simulink library "vmc"  (R2021b)
settings: Solver=VariableStepAuto  StartTime=0.0  StopTime=10.0  RelTol=1e-3
undefined symbols (not defined in the file or in its folder): AVMC_ACCDeltaTqIGain4OVRD_X_kph, AVMC_ACCDeltaTqIGain4OVRD_Y_mps2, AVMC_ACCDeltaTqIGain_X_kph, AVMC_ACCDeltaTqIGain_Y_mps2, AVMC_ACCDeltaTqPGain_X_kph, AVMC_ACCDeltaTqPGain_Y_kph, AVMC_ACCLongSteadyCtrl_X_kph, AVMC_ADSPosGFBDeltaTq_X_kph, AVMC_ADSPosGFBDeltaTq_Y_mps2, AVMC_AggressJerkPCT4AT_X_kph, AVMC_AggressJerkPCT_X_kph, AVMC_AggressLimitPCT4AT_X_kph, AVMC_AggressLimitPCT_X_kph, AVMC_CCLongSteadyCtrl_X_kph, AVMC_DISCDeltaTqIGain_X_kph, AVMC_DISCDeltaTqIGain_Y_mps2, AVMC_DISCDeltaTqPGain_X_kph, AVMC_DISCDeltaTqPGain_Y_kph, AVMC_ESCRegenOut_X_kph, AVMC_ESCRegenOut_Y_Deg, AVMC_ESCRegenOutEnSpd_X_Deg, AVMC_ISOAccLimit_X_mps, AVMC_ISODecLimit_X_mps, AVMC_ISOJerk_X_mps, AVMC_LatESCRegenOut_X_kph, AVMC_LatESCRegenOut_Y_Deg, AVMC_LongAccDeadZone_X_kph, AVMC_LongAccFiltTsforP2_X_Gps, AVMC_MCPresBaseTq_X_bar, AVMC_MSALongSteadyCtrl_X_kph, AVMC_MSAPedalOvrd_X_kph, AVMC_MSASpdBand_X_kph, AVMC_MSATqDownEndTq_X_kph, AVMC_MSATqDownTime_X_kph, AVMC_OPDDisSlideRate_X_Deg, AVMC_OVRD2ActSR2FCMCMD_X_mps2, AVMC_PedalTqRWhlRatio_X_Nm, AVMC_PedalTqRWhlRatio_Y_gps, AVMC_PedalTqRWhlSlipGain_X_rat, AVMC_PedalTqRWhlSlipGain_Y_kph, AVMC_PedalTqRWhSTRGGain_X_deg, AVMC_PedalTqRWhSTRGGain_Y_kph, AVMC_RDCDetectTime_X_kph, AVMC_RDCDetectTime_Y_pct, AVMC_RDCEnSlideRate_X_Deg, AVMC_RearWhlTqRatio_X_Nm, AVMC_RearWhlTqRatio_Y_gps, AVMC_RearWhlTqSlipGain_X_rat, AVMC_RearWhlTqSlipGain_Y_kph, AVMC_RearWhlTqSTRGGain_X_deg, AVMC_RearWhlTqSTRGGain_Y_kph, AVMC_ReqBrkJoinDecSR_X_mps2, AVMC_SoftJerkPCT_X_kph, AVMC_SoftLimitPCT_X_kph, AVMC_StESCYaw_X_kph, AVMC_StESCYaw_Y_Deg, AVMC_StESCYawCom_X_kph, AVMC_StESCYawCom_Y_Gps, AVMC_TMSpdBaseTq_X_rpm, AVMC_VehHoldDecCtrlTime2_X_kph ... (+411)
libraries: hcu_lib x108, simulink x82, tqr x1, simulink_extras x1
(part 14 of 14)

== stateflow chart vmc/VMC/VMC/SpeedCalculation/RollingAverage ==
  state LatAccelRollingAverage
    (default) -> (junction 2) : {VVMC_RollAveCount_enum = ONE_INT}
    LatAccelRollingAverage -> (junction 2)
    (junction 2) -> (junction 3) : {VVMC_RollAve_kph = ZERO_FLOAT}
    (junction 3) -> (junction 100) [order 1] : [VVMC_RollAveCount_enum < KVMC_RollAveLevel_enum]
    (junction 3) -> (junction 37) [order 2]
    (junction 100) -> (junction 5) : {% Memory
        |  VVMC_Memory_raw32[VVMC_RollAveCount_enum] = VINP_RawData_kph;
        |
        |  % Memory Shift Counter
        |  VVMC_ShiftCount_enum = ONE_INT}
    (junction 5) -> (junction 7) [order 2]
    (junction 5) -> (junction 6) [order 1] : [VVMC_ShiftCount_enum <= VVMC_RollAveCount_enum]
    (junction 7) -> (junction 8) : {% Rolling Average
        |  VVMC_RollAve_kph = VVMC_RollAve_kph / VVMC_RollAveCount_enum;
        |
        |  % Rolling Average Counter
        |  VVMC_RollAveCount_enum++}
    (junction 35) -> (junction 5) : {VVMC_ShiftCount_enum++}
    (junction 6) -> (junction 36) : {% Rolling Average Sum
        |  VVMC_RollAve_kph = VVMC_RollAve_kph + VVMC_Memory_raw32[VVMC_ShiftCount_enum];
        |  }
    (junction 36) -> (junction 35)
    (junction 37) -> (junction 76) [order 1] : [VVMC_RollAveCount_enum == KVMC_RollAveLevel_enum]
    (junction 76) -> (junction 47)
    (junction 37) -> (junction 60) [order 2]
    (junction 78) -> (junction 76)
    (junction 47) -> (junction 30) : {% Memory
        |  VVMC_Memory_raw32[VVMC_RollAveCount_enum] = VINP_RawData_kph;
        |
        |  % Memory Shift Counter
        |  VVMC_ShiftCount_enum = ONE_INT;
        | }
    (junction 60) -> (junction 62) [order 1] : [VVMC_RollAveCount_enum > KVMC_RollAveLevel_enum]
    (junction 60) -> (junction 39) [order 2]
    (junction 62) -> (junction 66) : {VVMC_MemoryShiftCount_enum = ONE_INT}
    (junction 30) -> (junction 48) [order 2]
    (junction 30) -> (junction 22) [order 1] : [VVMC_ShiftCount_enum <= VVMC_RollAveCount_enum]
    (junction 48) -> (junction 45) : {% Rolling Average
        |  VVMC_RollAve_kph = VVMC_RollAve_kph / VVMC_RollAveCount_enum;
        |
        |  % Memory Shift Counter
        |  VVMC_ShiftCount_enum = ONE_INT}
    (junction 14) -> (junction 30) : {VVMC_ShiftCount_enum++}
    (junction 22) -> (junction 25) : {% Rolling Average Sum
        |  VVMC_RollAve_kph = VVMC_RollAve_kph + VVMC_Memory_raw32[VVMC_ShiftCount_enum]}
    (junction 66) -> (junction 82) [order 2]
    (junction 66) -> (junction 69) [order 1] : [VVMC_MemoryShiftCount_enum < VVMC_RollAveCount_enum]
    (junction 82) -> (junction 80) : {VVMC_RollAveCount_enum = KVMC_RollAveLevel_enum}
    (junction 73) -> (junction 66) : {VVMC_MemoryShiftCount_enum++}
    (junction 69) -> (junction 71) : {VVMC_Memory_raw32[VVMC_MemoryShiftCount_enum] =...
        |  VVMC_Memory_raw32[VVMC_RollAveCount_enum - KVMC_RollAveLevel_enum + VVMC_MemoryShiftCount_enum]}
    (junction 25) -> (junction 14)
    (junction 71) -> (junction 73)
    (junction 80) -> (junction 78)
    (junction 45) -> (junction 39) [order 2]
    (junction 45) -> (junction 15) [order 1] : [VVMC_ShiftCount_enum < VVMC_RollAveCount_enum]
    (junction 41) -> (junction 45) : { VVMC_ShiftCount_enum++}
    (junction 15) -> (junction 38) : {% Gy Memory Shift
        |  VVMC_Memory_raw32[VVMC_ShiftCount_enum] = VVMC_Memory_raw32[VVMC_ShiftCount_enum + ONE_INT]}
    (junction 38) -> (junction 41)
  data: KVMC_RollAveLevel_enum input uint8; VVMC_ShiftCount_enum local uint8; VVMC_RollAveCount_enum local uint8; VVMC_Memory_raw32 local single size=256; ZERO_FLOAT input single; ONE_INT input uint8; VVMC_RollAve_kph output single; VINP_RawData_kph input single; VVMC_MemoryShiftCount_enum local uint8

== stateflow chart vmc/VMC/VMC/SafetyControl/WheelSpeedRollingAverage/RollingAverage ==
  state LatAccelRollingAverage
    (default) -> (junction 2) : {VVMC_RollAveCount_enum = ONE_INT}
    LatAccelRollingAverage -> (junction 2)
    (junction 2) -> (junction 3) : {VVMC_LFWhlSpeedRollAveRaw_kph = ZERO_FLOAT}
    (junction 3) -> (junction 100) [order 1] : [VVMC_RollAveCount_enum < KVMC_WhlSpdRollAveLevel_enum]
    (junction 3) -> (junction 37) [order 2]
    (junction 100) -> (junction 5) : {% Memory
        |  VVMC_Memory_raw32[VVMC_RollAveCount_enum] = VINP_LFRawWhlSpeed_kph;
        |
        |  % Memory Shift Counter
        |  VVMC_ShiftCount_enum = ONE_INT}
    (junction 5) -> (junction 7) [order 2]
    (junction 5) -> (junction 6) [order 1] : [VVMC_ShiftCount_enum <= VVMC_RollAveCount_enum]
    (junction 7) -> (junction 8) : {% Rolling Average
        |  VVMC_LFWhlSpeedRollAveRaw_kph = VVMC_LFWhlSpeedRollAveRaw_kph / VVMC_RollAveCount_enum;
        |
        |  % Rolling Average Counter
        |  VVMC_RollAveCount_enum++}
    (junction 35) -> (junction 5) : {VVMC_ShiftCount_enum++}
    (junction 6) -> (junction 36) : {% Rolling Average Sum
        |  VVMC_LFWhlSpeedRollAveRaw_kph = VVMC_LFWhlSpeedRollAveRaw_kph + VVMC_Memory_raw32[VVMC_ShiftCount_enum];
        |  }
    (junction 36) -> (junction 35)
    (junction 37) -> (junction 76) [order 1] : [VVMC_RollAveCount_enum == KVMC_WhlSpdRollAveLevel_enum]
    (junction 76) -> (junction 47)
    (junction 37) -> (junction 60) [order 2]
    (junction 78) -> (junction 76)
    (junction 47) -> (junction 30) : {% Memory
        |  VVMC_Memory_raw32[VVMC_RollAveCount_enum] = VINP_LFRawWhlSpeed_kph;
        |
        |  % Memory Shift Counter
        |  VVMC_ShiftCount_enum = ONE_INT;
        | }
    (junction 60) -> (junction 62) [order 1] : [VVMC_RollAveCount_enum > KVMC_WhlSpdRollAveLevel_enum]
    (junction 60) -> (junction 39) [order 2]
    (junction 62) -> (junction 66) : {VVMC_MemoryShiftCount_enum = ONE_INT}
    (junction 30) -> (junction 48) [order 2]
    (junction 30) -> (junction 22) [order 1] : [VVMC_ShiftCount_enum <= VVMC_RollAveCount_enum]
    (junction 48) -> (junction 45) : {% Rolling Average
        |  VVMC_LFWhlSpeedRollAveRaw_kph = VVMC_LFWhlSpeedRollAveRaw_kph / VVMC_RollAveCount_enum;
        |
        |  % Memory Shift Counter
        |  VVMC_ShiftCount_enum = ONE_INT}
    (junction 14) -> (junction 30) : {VVMC_ShiftCount_enum++}
    (junction 22) -> (junction 25) : {% Rolling Average Sum
        |  VVMC_LFWhlSpeedRollAveRaw_kph = VVMC_LFWhlSpeedRollAveRaw_kph + VVMC_Memory_raw32[VVMC_ShiftCount_enum]}
    (junction 66) -> (junction 82) [order 2]
    (junction 66) -> (junction 69) [order 1] : [VVMC_MemoryShiftCount_enum < VVMC_RollAveCount_enum]
    (junction 82) -> (junction 80) : {VVMC_RollAveCount_enum = KVMC_WhlSpdRollAveLevel_enum}
    (junction 73) -> (junction 66) : {VVMC_MemoryShiftCount_enum++}
    (junction 69) -> (junction 71) : {VVMC_Memory_raw32[VVMC_MemoryShiftCount_enum] =...
        |  VVMC_Memory_raw32[VVMC_RollAveCount_enum - KVMC_WhlSpdRollAveLevel_enum + VVMC_MemoryShiftCount_enum]}
    (junction 25) -> (junction 14)
    (junction 71) -> (junction 73)
    (junction 80) -> (junction 78)
    (junction 45) -> (junction 39) [order 2]
    (junction 45) -> (junction 15) [order 1] : [VVMC_ShiftCount_enum < VVMC_RollAveCount_enum]
    (junction 41) -> (junction 45) : { VVMC_ShiftCount_enum++}
    (junction 15) -> (junction 38) : {% Gy Memory Shift
        |  VVMC_Memory_raw32[VVMC_ShiftCount_enum] = VVMC_Memory_raw32[VVMC_ShiftCount_enum + ONE_INT]}
    (junction 38) -> (junction 41)
  data: KVMC_WhlSpdRollAveLevel_enum input uint8; VVMC_ShiftCount_enum local uint8; VVMC_RollAveCount_enum local uint8; VVMC_Memory_raw32 local single size=256; ZERO_FLOAT input single; ONE_INT input uint8; VINP_LFRawWhlSpeed_kph input single; VVMC_MemoryShiftCount_enum local uint8; VVMC_LFWhlSpeedRollAveRaw_kph output single

== stateflow chart vmc/VMC/VMC/SafetyControl/WheelSpeedRollingAverage/RollingAverage1 ==
  state LatAccelRollingAverage
    (default) -> (junction 2) : {VVMC_RollAveCount_enum = ONE_INT}
    LatAccelRollingAverage -> (junction 2)
    (junction 2) -> (junction 3) : {VVMC_RFWhlSpeedRollAveRaw_kph = ZERO_FLOAT}
    (junction 3) -> (junction 100) [order 1] : [VVMC_RollAveCount_enum < KVMC_WhlSpdRollAveLevel_enum]
    (junction 3) -> (junction 37) [order 2]
    (junction 100) -> (junction 5) : {% Memory
        |  VVMC_Memory_raw32[VVMC_RollAveCount_enum] = VINP_RFRawWhlSpeed_kph;
        |
        |  % Memory Shift Counter
        |  VVMC_ShiftCount_enum = ONE_INT}
    (junction 5) -> (junction 7) [order 2]
    (junction 5) -> (junction 6) [order 1] : [VVMC_ShiftCount_enum <= VVMC_RollAveCount_enum]
    (junction 7) -> (junction 8) : {% Rolling Average
        |  VVMC_RFWhlSpeedRollAveRaw_kph = VVMC_RFWhlSpeedRollAveRaw_kph / VVMC_RollAveCount_enum;
        |
        |  % Rolling Average Counter
        |  VVMC_RollAveCount_enum++}
    (junction 35) -> (junction 5) : {VVMC_ShiftCount_enum++}
    (junction 6) -> (junction 36) : {% Rolling Average Sum
        |  VVMC_RFWhlSpeedRollAveRaw_kph = VVMC_RFWhlSpeedRollAveRaw_kph + VVMC_Memory_raw32[VVMC_ShiftCount_enum];
        |  }
    (junction 36) -> (junction 35)
    (junction 37) -> (junction 76) [order 1] : [VVMC_RollAveCount_enum == KVMC_WhlSpdRollAveLevel_enum]
    (junction 76) -> (junction 47)
    (junction 37) -> (junction 60) [order 2]
    (junction 78) -> (junction 76)
    (junction 47) -> (junction 30) : {% Memory
        |  VVMC_Memory_raw32[VVMC_RollAveCount_enum] = VINP_RFRawWhlSpeed_kph;
        |
        |  % Memory Shift Counter
        |  VVMC_ShiftCount_enum = ONE_INT;
        | }
    (junction 60) -> (junction 62) [order 1] : [VVMC_RollAveCount_enum > KVMC_WhlSpdRollAveLevel_enum]
    (junction 60) -> (junction 39) [order 2]
    (junction 62) -> (junction 66) : {VVMC_MemoryShiftCount_enum = ONE_INT}
    (junction 30) -> (junction 48) [order 2]
    (junction 30) -> (junction 22) [order 1] : [VVMC_ShiftCount_enum <= VVMC_RollAveCount_enum]
    (junction 48) -> (junction 45) : {% Rolling Average
        |  VVMC_RFWhlSpeedRollAveRaw_kph = VVMC_RFWhlSpeedRollAveRaw_kph / VVMC_RollAveCount_enum;
        |
        |  % Memory Shift Counter
        |  VVMC_ShiftCount_enum = ONE_INT}
    (junction 14) -> (junction 30) : {VVMC_ShiftCount_enum++}
    (junction 22) -> (junction 25) : {% Rolling Average Sum
        |  VVMC_RFWhlSpeedRollAveRaw_kph = VVMC_RFWhlSpeedRollAveRaw_kph + VVMC_Memory_raw32[VVMC_ShiftCount_enum]}
    (junction 66) -> (junction 82) [order 2]
    (junction 66) -> (junction 69) [order 1] : [VVMC_MemoryShiftCount_enum < VVMC_RollAveCount_enum]
    (junction 82) -> (junction 80) : {VVMC_RollAveCount_enum = KVMC_WhlSpdRollAveLevel_enum}
    (junction 73) -> (junction 66) : {VVMC_MemoryShiftCount_enum++}
    (junction 69) -> (junction 71) : {VVMC_Memory_raw32[VVMC_MemoryShiftCount_enum] =...
        |  VVMC_Memory_raw32[VVMC_RollAveCount_enum - KVMC_WhlSpdRollAveLevel_enum + VVMC_MemoryShiftCount_enum]}
    (junction 25) -> (junction 14)
    (junction 71) -> (junction 73)
    (junction 80) -> (junction 78)
    (junction 45) -> (junction 39) [order 2]
    (junction 45) -> (junction 15) [order 1] : [VVMC_ShiftCount_enum < VVMC_RollAveCount_enum]
    (junction 41) -> (junction 45) : { VVMC_ShiftCount_enum++}
    (junction 15) -> (junction 38) : {% Gy Memory Shift
        |  VVMC_Memory_raw32[VVMC_ShiftCount_enum] = VVMC_Memory_raw32[VVMC_ShiftCount_enum + ONE_INT]}
    (junction 38) -> (junction 41)
  data: KVMC_WhlSpdRollAveLevel_enum input uint8; VVMC_ShiftCount_enum local uint8; VVMC_RollAveCount_enum local uint8; VVMC_Memory_raw32 local single size=256; ZERO_FLOAT input single; ONE_INT input uint8; VINP_RFRawWhlSpeed_kph input single; VVMC_MemoryShiftCount_enum local uint8; VVMC_RFWhlSpeedRollAveRaw_kph output single

== stateflow chart vmc/VMC/VMC/SafetyControl/WheelSpeedRollingAverage/RollingAverage2 ==
  state LatAccelRollingAverage
    (default) -> (junction 2) : {VVMC_RollAveCount_enum = ONE_INT}
    LatAccelRollingAverage -> (junction 2)
    (junction 2) -> (junction 3) : {VVMC_LRWhlSpeedRollAveRaw_kph = ZERO_FLOAT}
    (junction 3) -> (junction 100) [order 1] : [VVMC_RollAveCount_enum < KVMC_WhlSpdRollAveLevel_enum]
    (junction 3) -> (junction 37) [order 2]
    (junction 100) -> (junction 5) : {% Memory
        |  VVMC_Memory_raw32[VVMC_RollAveCount_enum] = VINP_LRRawWhlSpeed_kph;
        |
        |  % Memory Shift Counter
        |  VVMC_ShiftCount_enum = ONE_INT}
    (junction 5) -> (junction 7) [order 2]
    (junction 5) -> (junction 6) [order 1] : [VVMC_ShiftCount_enum <= VVMC_RollAveCount_enum]
    (junction 7) -> (junction 8) : {% Rolling Average
        |  VVMC_LRWhlSpeedRollAveRaw_kph = VVMC_LRWhlSpeedRollAveRaw_kph / VVMC_RollAveCount_enum;
        |
        |  % Rolling Average Counter
        |  VVMC_RollAveCount_enum++}
    (junction 35) -> (junction 5) : {VVMC_ShiftCount_enum++}
    (junction 6) -> (junction 36) : {% Rolling Average Sum
        |  VVMC_LRWhlSpeedRollAveRaw_kph = VVMC_LRWhlSpeedRollAveRaw_kph + VVMC_Memory_raw32[VVMC_ShiftCount_enum];
        |  }
    (junction 36) -> (junction 35)
    (junction 37) -> (junction 76) [order 1] : [VVMC_RollAveCount_enum == KVMC_WhlSpdRollAveLevel_enum]
    (junction 76) -> (junction 47)
    (junction 37) -> (junction 60) [order 2]
    (junction 78) -> (junction 76)
    (junction 47) -> (junction 30) : {% Memory
        |  VVMC_Memory_raw32[VVMC_RollAveCount_enum] = VINP_LRRawWhlSpeed_kph;
        |
        |  % Memory Shift Counter
        |  VVMC_ShiftCount_enum = ONE_INT;
        | }
    (junction 60) -> (junction 62) [order 1] : [VVMC_RollAveCount_enum > KVMC_WhlSpdRollAveLevel_enum]
    (junction 60) -> (junction 39) [order 2]
    (junction 62) -> (junction 66) : {VVMC_MemoryShiftCount_enum = ONE_INT}
    (junction 30) -> (junction 48) [order 2]
    (junction 30) -> (junction 22) [order 1] : [VVMC_ShiftCount_enum <= VVMC_RollAveCount_enum]
    (junction 48) -> (junction 45) : {% Rolling Average
        |  VVMC_LRWhlSpeedRollAveRaw_kph = VVMC_LRWhlSpeedRollAveRaw_kph / VVMC_RollAveCount_enum;
        |
        |  % Memory Shift Counter
        |  VVMC_ShiftCount_enum = ONE_INT}
    (junction 14) -> (junction 30) : {VVMC_ShiftCount_enum++}
    (junction 22) -> (junction 25) : {% Rolling Average Sum
        |  VVMC_LRWhlSpeedRollAveRaw_kph = VVMC_LRWhlSpeedRollAveRaw_kph + VVMC_Memory_raw32[VVMC_ShiftCount_enum]}
    (junction 66) -> (junction 82) [order 2]
    (junction 66) -> (junction 69) [order 1] : [VVMC_MemoryShiftCount_enum < VVMC_RollAveCount_enum]
    (junction 82) -> (junction 80) : {VVMC_RollAveCount_enum = KVMC_WhlSpdRollAveLevel_enum}
    (junction 73) -> (junction 66) : {VVMC_MemoryShiftCount_enum++}
    (junction 69) -> (junction 71) : {VVMC_Memory_raw32[VVMC_MemoryShiftCount_enum] =...
        |  VVMC_Memory_raw32[VVMC_RollAveCount_enum - KVMC_WhlSpdRollAveLevel_enum + VVMC_MemoryShiftCount_enum]}
    (junction 25) -> (junction 14)
    (junction 71) -> (junction 73)
    (junction 80) -> (junction 78)
    (junction 45) -> (junction 39) [order 2]
    (junction 45) -> (junction 15) [order 1] : [VVMC_ShiftCount_enum < VVMC_RollAveCount_enum]
    (junction 41) -> (junction 45) : { VVMC_ShiftCount_enum++}
    (junction 15) -> (junction 38) : {% Gy Memory Shift
        |  VVMC_Memory_raw32[VVMC_ShiftCount_enum] = VVMC_Memory_raw32[VVMC_ShiftCount_enum + ONE_INT]}
    (junction 38) -> (junction 41)
  data: KVMC_WhlSpdRollAveLevel_enum input uint8; VVMC_ShiftCount_enum local uint8; VVMC_RollAveCount_enum local uint8; VVMC_Memory_raw32 local single size=256; ZERO_FLOAT input single; ONE_INT input uint8; VINP_LRRawWhlSpeed_kph input single; VVMC_MemoryShiftCount_enum local uint8; VVMC_LRWhlSpeedRollAveRaw_kph output single

== stateflow chart vmc/VMC/VMC/SafetyControl/WheelSpeedRollingAverage/RollingAverage3 ==
  state LatAccelRollingAverage
    (default) -> (junction 2) : {VVMC_RollAveCount_enum = ONE_INT}
    LatAccelRollingAverage -> (junction 2)
    (junction 2) -> (junction 3) : {VVMC_RRWhlSpeedRollAveRaw_kph = ZERO_FLOAT}
    (junction 3) -> (junction 100) [order 1] : [VVMC_RollAveCount_enum < KVMC_WhlSpdRollAveLevel_enum]
    (junction 3) -> (junction 37) [order 2]
    (junction 100) -> (junction 5) : {% Memory
        |  VVMC_Memory_raw32[VVMC_RollAveCount_enum] = VINP_RRRawWhlSpeed_kph;
        |
        |  % Memory Shift Counter
        |  VVMC_ShiftCount_enum = ONE_INT}
    (junction 5) -> (junction 7) [order 2]
    (junction 5) -> (junction 6) [order 1] : [VVMC_ShiftCount_enum <= VVMC_RollAveCount_enum]
    (junction 7) -> (junction 8) : {% Rolling Average
        |  VVMC_RRWhlSpeedRollAveRaw_kph = VVMC_RRWhlSpeedRollAveRaw_kph / VVMC_RollAveCount_enum;
        |
        |  % Rolling Average Counter
        |  VVMC_RollAveCount_enum++}
    (junction 35) -> (junction 5) : {VVMC_ShiftCount_enum++}
    (junction 6) -> (junction 36) : {% Rolling Average Sum
        |  VVMC_RRWhlSpeedRollAveRaw_kph = VVMC_RRWhlSpeedRollAveRaw_kph + VVMC_Memory_raw32[VVMC_ShiftCount_enum];
        |  }
    (junction 36) -> (junction 35)
    (junction 37) -> (junction 76) [order 1] : [VVMC_RollAveCount_enum == KVMC_WhlSpdRollAveLevel_enum]
    (junction 76) -> (junction 47)
    (junction 37) -> (junction 60) [order 2]
    (junction 78) -> (junction 76)
    (junction 47) -> (junction 30) : {% Memory
        |  VVMC_Memory_raw32[VVMC_RollAveCount_enum] = VINP_RRRawWhlSpeed_kph;
        |
        |  % Memory Shift Counter
        |  VVMC_ShiftCount_enum = ONE_INT;
        | }
    (junction 60) -> (junction 62) [order 1] : [VVMC_RollAveCount_enum > KVMC_WhlSpdRollAveLevel_enum]
    (junction 60) -> (junction 39) [order 2]
    (junction 62) -> (junction 66) : {VVMC_MemoryShiftCount_enum = ONE_INT}
    (junction 30) -> (junction 48) [order 2]
    (junction 30) -> (junction 22) [order 1] : [VVMC_ShiftCount_enum <= VVMC_RollAveCount_enum]
    (junction 48) -> (junction 45) : {% Rolling Average
        |  VVMC_RRWhlSpeedRollAveRaw_kph = VVMC_RRWhlSpeedRollAveRaw_kph / VVMC_RollAveCount_enum;
        |
        |  % Memory Shift Counter
        |  VVMC_ShiftCount_enum = ONE_INT}
    (junction 14) -> (junction 30) : {VVMC_ShiftCount_enum++}
    (junction 22) -> (junction 25) : {% Rolling Average Sum
        |  VVMC_RRWhlSpeedRollAveRaw_kph = VVMC_RRWhlSpeedRollAveRaw_kph + VVMC_Memory_raw32[VVMC_ShiftCount_enum]}
    (junction 66) -> (junction 82) [order 2]
    (junction 66) -> (junction 69) [order 1] : [VVMC_MemoryShiftCount_enum < VVMC_RollAveCount_enum]
    (junction 82) -> (junction 80) : {VVMC_RollAveCount_enum = KVMC_WhlSpdRollAveLevel_enum}
    (junction 73) -> (junction 66) : {VVMC_MemoryShiftCount_enum++}
    (junction 69) -> (junction 71) : {VVMC_Memory_raw32[VVMC_MemoryShiftCount_enum] =...
        |  VVMC_Memory_raw32[VVMC_RollAveCount_enum - KVMC_WhlSpdRollAveLevel_enum + VVMC_MemoryShiftCount_enum]}
    (junction 25) -> (junction 14)
    (junction 71) -> (junction 73)
    (junction 80) -> (junction 78)
    (junction 45) -> (junction 39) [order 2]
    (junction 45) -> (junction 15) [order 1] : [VVMC_ShiftCount_enum < VVMC_RollAveCount_enum]
    (junction 41) -> (junction 45) : { VVMC_ShiftCount_enum++}
    (junction 15) -> (junction 38) : {% Gy Memory Shift
        |  VVMC_Memory_raw32[VVMC_ShiftCount_enum] = VVMC_Memory_raw32[VVMC_ShiftCount_enum + ONE_INT]}
    (junction 38) -> (junction 41)
  data: KVMC_WhlSpdRollAveLevel_enum input uint8; VVMC_ShiftCount_enum local uint8; VVMC_RollAveCount_enum local uint8; VVMC_Memory_raw32 local single size=256; ZERO_FLOAT input single; ONE_INT input uint8; VINP_RRRawWhlSpeed_kph input single; VVMC_MemoryShiftCount_enum local uint8; VVMC_RRWhlSpeedRollAveRaw_kph output single

== stateflow chart vmc/VMC/VMC/IMU/IMU sensing result /RollingAverage4 ==
  state RollingAverage
    (default) -> (junction 2) : {VVMC_RollAveCount_enum = ONE_INT}
    RollingAverage -> (junction 2)
    (junction 2) -> (junction 3) : {VVMC_RollAve_raw32 = ZERO_FLOAT}
    (junction 3) -> (junction 100) [order 1] : [VVMC_RollAveCount_enum < KVMC_RollAveLevel_enum]
    (junction 3) -> (junction 37) [order 2]
    (junction 100) -> (junction 5) : {% Memory
        |  VVMC_Memory_raw32[VVMC_RollAveCount_enum] = VINP_INPData_raw32;
        |
        |  % Memory Shift Counter
        |  VVMC_ShiftCount_enum = ONE_INT}
    (junction 5) -> (junction 7) [order 2]
    (junction 5) -> (junction 6) [order 1] : [VVMC_ShiftCount_enum <= VVMC_RollAveCount_enum]
    (junction 7) -> (junction 8) : {% Rolling Average
        |  VVMC_RollAve_raw32 = VVMC_RollAve_raw32 / VVMC_RollAveCount_enum;
        |
        |  % Rolling Average Counter
        |  VVMC_RollAveCount_enum++}
    (junction 35) -> (junction 5) : {VVMC_ShiftCount_enum++}
    (junction 6) -> (junction 36) : {% Rolling Average Sum
        |  VVMC_RollAve_raw32 = VVMC_RollAve_raw32 + VVMC_Memory_raw32[VVMC_ShiftCount_enum];
        |  }
    (junction 36) -> (junction 35)
    (junction 37) -> (junction 76) [order 1] : [VVMC_RollAveCount_enum == KVMC_RollAveLevel_enum]
    (junction 76) -> (junction 47)
    (junction 37) -> (junction 60) [order 2]
    (junction 78) -> (junction 76)
    (junction 47) -> (junction 30) : {% Memory
        |  VVMC_Memory_raw32[VVMC_RollAveCount_enum] = VINP_INPData_raw32;
        |
        |  % Memory Shift Counter
        |  VVMC_ShiftCount_enum = ONE_INT;
        | }
    (junction 60) -> (junction 62) [order 1] : [VVMC_RollAveCount_enum > KVMC_RollAveLevel_enum]
    (junction 60) -> (junction 39) [order 2]
    (junction 62) -> (junction 66) : {VVMC_MemoryShiftCount_enum = ONE_INT}
    (junction 30) -> (junction 48) [order 2]
    (junction 30) -> (junction 22) [order 1] : [VVMC_ShiftCount_enum <= VVMC_RollAveCount_enum]
    (junction 48) -> (junction 45) : {% Rolling Average
        |  VVMC_RollAve_raw32 = VVMC_RollAve_raw32 / VVMC_RollAveCount_enum;
        |
        |  % Memory Shift Counter
        |  VVMC_ShiftCount_enum = ONE_INT}
    (junction 14) -> (junction 30) : {VVMC_ShiftCount_enum++}
    (junction 22) -> (junction 25) : {% Rolling Average Sum
        |  VVMC_RollAve_raw32 = VVMC_RollAve_raw32 + VVMC_Memory_raw32[VVMC_ShiftCount_enum]}
    (junction 66) -> (junction 82) [order 2]
    (junction 66) -> (junction 69) [order 1] : [VVMC_MemoryShiftCount_enum < VVMC_RollAveCount_enum]
    (junction 82) -> (junction 80) : {VVMC_RollAveCount_enum = KVMC_RollAveLevel_enum}
    (junction 73) -> (junction 66) : {VVMC_MemoryShiftCount_enum++}
    (junction 69) -> (junction 71) : {VVMC_Memory_raw32[VVMC_MemoryShiftCount_enum] =...
        |  VVMC_Memory_raw32[VVMC_RollAveCount_enum - KVMC_RollAveLevel_enum + VVMC_MemoryShiftCount_enum]}
    (junction 25) -> (junction 14)
    (junction 71) -> (junction 73)
    (junction 80) -> (junction 78)
    (junction 45) -> (junction 39) [order 2]
    (junction 45) -> (junction 15) [order 1] : [VVMC_ShiftCount_enum < VVMC_RollAveCount_enum]
    (junction 41) -> (junction 45) : { VVMC_ShiftCount_enum++}
    (junction 15) -> (junction 38) : {% Gy Memory Shift
        |  VVMC_Memory_raw32[VVMC_ShiftCount_enum] = VVMC_Memory_raw32[VVMC_ShiftCount_enum + ONE_INT]}
    (junction 38) -> (junction 41)
  data: KVMC_RollAveLevel_enum input uint8; VVMC_ShiftCount_enum local uint8; VVMC_RollAveCount_enum local uint8; VVMC_Memory_raw32 local single size=256; ZERO_FLOAT input single; ONE_INT input uint8; VVMC_RollAve_raw32 output single; VINP_INPData_raw32 input single; VVMC_MemoryShiftCount_enum local uint8

== stateflow chart vmc/VMC/VMC/IMU/IMU sensing result /RollingAverage5 ==
  state RollingAverage
    (default) -> (junction 2) : {VVMC_RollAveCount_enum = ONE_INT}
    RollingAverage -> (junction 2)
    (junction 2) -> (junction 3) : {VVMC_RollAve_raw32 = ZERO_FLOAT}
    (junction 3) -> (junction 100) [order 1] : [VVMC_RollAveCount_enum < KVMC_RollAveLevel_enum]
    (junction 3) -> (junction 37) [order 2]
    (junction 100) -> (junction 5) : {% Memory
        |  VVMC_Memory_raw32[VVMC_RollAveCount_enum] = VINP_INPData_raw32;
        |
        |  % Memory Shift Counter
        |  VVMC_ShiftCount_enum = ONE_INT}
    (junction 5) -> (junction 7) [order 2]
    (junction 5) -> (junction 6) [order 1] : [VVMC_ShiftCount_enum <= VVMC_RollAveCount_enum]
    (junction 7) -> (junction 8) : {% Rolling Average
        |  VVMC_RollAve_raw32 = VVMC_RollAve_raw32 / VVMC_RollAveCount_enum;
        |
        |  % Rolling Average Counter
        |  VVMC_RollAveCount_enum++}
    (junction 35) -> (junction 5) : {VVMC_ShiftCount_enum++}
    (junction 6) -> (junction 36) : {% Rolling Average Sum
        |  VVMC_RollAve_raw32 = VVMC_RollAve_raw32 + VVMC_Memory_raw32[VVMC_ShiftCount_enum];
        |  }
    (junction 36) -> (junction 35)
    (junction 37) -> (junction 76) [order 1] : [VVMC_RollAveCount_enum == KVMC_RollAveLevel_enum]
    (junction 76) -> (junction 47)
    (junction 37) -> (junction 60) [order 2]
    (junction 78) -> (junction 76)
    (junction 47) -> (junction 30) : {% Memory
        |  VVMC_Memory_raw32[VVMC_RollAveCount_enum] = VINP_INPData_raw32;
        |
        |  % Memory Shift Counter
        |  VVMC_ShiftCount_enum = ONE_INT;
        | }
    (junction 60) -> (junction 62) [order 1] : [VVMC_RollAveCount_enum > KVMC_RollAveLevel_enum]
    (junction 60) -> (junction 39) [order 2]
    (junction 62) -> (junction 66) : {VVMC_MemoryShiftCount_enum = ONE_INT}
    (junction 30) -> (junction 48) [order 2]
    (junction 30) -> (junction 22) [order 1] : [VVMC_ShiftCount_enum <= VVMC_RollAveCount_enum]
    (junction 48) -> (junction 45) : {% Rolling Average
        |  VVMC_RollAve_raw32 = VVMC_RollAve_raw32 / VVMC_RollAveCount_enum;
        |
        |  % Memory Shift Counter
        |  VVMC_ShiftCount_enum = ONE_INT}
    (junction 14) -> (junction 30) : {VVMC_ShiftCount_enum++}
    (junction 22) -> (junction 25) : {% Rolling Average Sum
        |  VVMC_RollAve_raw32 = VVMC_RollAve_raw32 + VVMC_Memory_raw32[VVMC_ShiftCount_enum]}
    (junction 66) -> (junction 82) [order 2]
    (junction 66) -> (junction 69) [order 1] : [VVMC_MemoryShiftCount_enum < VVMC_RollAveCount_enum]
    (junction 82) -> (junction 80) : {VVMC_RollAveCount_enum = KVMC_RollAveLevel_enum}
    (junction 73) -> (junction 66) : {VVMC_MemoryShiftCount_enum++}
    (junction 69) -> (junction 71) : {VVMC_Memory_raw32[VVMC_MemoryShiftCount_enum] =...
        |  VVMC_Memory_raw32[VVMC_RollAveCount_enum - KVMC_RollAveLevel_enum + VVMC_MemoryShiftCount_enum]}
    (junction 25) -> (junction 14)
    (junction 71) -> (junction 73)
    (junction 80) -> (junction 78)
    (junction 45) -> (junction 39) [order 2]
    (junction 45) -> (junction 15) [order 1] : [VVMC_ShiftCount_enum < VVMC_RollAveCount_enum]
    (junction 41) -> (junction 45) : { VVMC_ShiftCount_enum++}
    (junction 15) -> (junction 38) : {% Gy Memory Shift
        |  VVMC_Memory_raw32[VVMC_ShiftCount_enum] = VVMC_Memory_raw32[VVMC_ShiftCount_enum + ONE_INT]}
    (junction 38) -> (junction 41)
  data: KVMC_RollAveLevel_enum input uint8; VVMC_ShiftCount_enum local uint8; VVMC_RollAveCount_enum local uint8; VVMC_Memory_raw32 local single size=256; ZERO_FLOAT input single; ONE_INT input uint8; VVMC_RollAve_raw32 output single; VINP_INPData_raw32 input single; VVMC_MemoryShiftCount_enum local uint8

== stateflow chart vmc/VMC/VMC/SPD2ACC/VVMC_DISReqAcc_mps2/ConstantSpeedControl ==
  state ConstantSpeedControl
    (default) -> (junction 2) : {SpdCtrlFlag = 0;
        |  ReqAccel = 0}
    ConstantSpeedControl -> (junction 2)
    (junction 2) -> (junction 6) [order 1] : [DeltaSpeed >= KVMC_SpdCtrlEnBand_kph && SpdCtrlFlag == 0 && ZeroDeltaSpd]
    (junction 2) -> (junction 16) [order 2]
    (junction 6) -> (junction 8) : {SpdCtrlFlag = 1;
        |  ReqAccel = MINUSONE_FLOAT * KVMC_SpdCtrlReqAccel_mps2}
    (junction 16) -> (junction 15) [order 1] : [DeltaSpeed <= MINUSONE_FLOAT * KVMC_SpdCtrlEnBand_kph && SpdCtrlFlag == 0 && ZeroDeltaSpd]
    (junction 16) -> (junction 20) [order 2]
    (junction 15) -> (junction 12) : {SpdCtrlFlag = 1;
        |  ReqAccel = KVMC_SpdCtrlReqAccel_mps2}
    (junction 20) -> (junction 18) [order 1] : [ZeroDeltaSpd && SpdCtrlFlag == 1]
    (junction 18) -> (junction 24) [order 1] : [ReqAccel > ZERO_FLOAT]
    (junction 24) -> (junction 26) [order 1] : [DeltaSpeed >= KVMC_SpdCtrlDisBand_kph]
    (junction 20) -> (junction 42) [order 2] : {SpdCtrlFlag = 0;
        |  ReqAccel = ZERO_FLOAT}
    (junction 18) -> (junction 40) [order 2]
    (junction 24) -> (junction 30) [order 2] : {SpdCtrlFlag = 1;
        |  ReqAccel = KVMC_SpdCtrlReqAccel_mps2}
    (junction 26) -> (junction 28) : {SpdCtrlFlag = 0;
        |  ReqAccel = ZERO_FLOAT}
    (junction 40) -> (junction 37) [order 1] : [ReqAccel < ZERO_FLOAT]
    (junction 37) -> (junction 33) [order 1] : [DeltaSpeed <= MINUSONE_FLOAT * KVMC_SpdCtrlDisBand_kph]
    (junction 40) -> (junction 49) [order 2]
    (junction 37) -> (junction 35) [order 2] : {SpdCtrlFlag = 1;
        |  ReqAccel = MINUSONE_FLOAT * KVMC_SpdCtrlReqAccel_mps2}
    (junction 33) -> (junction 38) : {SpdCtrlFlag = 0;
        |  ReqAccel = ZERO_FLOAT}
  data: ZeroDeltaSpd input; DeltaSpeed input single; SpdCtrlFlag local boolean; ReqAccel output single; KVMC_SpdCtrlEnBand_kph input single; KVMC_SpdCtrlDisBand_kph input single; MINUSONE_FLOAT input single; KVMC_SpdCtrlReqAccel_mps2 input single; ZERO_FLOAT input single

== stateflow chart vmc/VMC/VMC/SafetyControl/SafetyControlJudgement/FrontRearSlipRatio/FrontRearSlipRatioJudgement ==
  state FrontRearSlipRatioJudgement
    (default) -> (junction 14) : {VVMC_FrontRearSlipRatioCtrl_flg = FALSE;
        |  VVMC_FrontAxleWhlSpeedAve_kph = ZERO_FLOAT;
        |  VVMC_RearAxleWhlSpeedAve_kph = ZERO_FLOAT}
    FrontRearSlipRatioJudgement -> (junction 14)
    (junction 14) -> (junction 41) [order 1] : [VINP_LFRawWhlSpeedV_flg == TRUE ||...
        |  VINP_RFRawWhlSpeedV_flg == TRUE]
    (junction 41) -> (junction 69) [order 1] : [VINP_LFRawWhlSpeedV_flg == TRUE &&...
        |  VINP_RFRawWhlSpeedV_flg == TRUE]
    (junction 14) -> (junction 54) [order 2] : {VVMC_FrontAxleWhlSpeedAve_kph =...
        | (VVMC_LFWhlSpeedRollAve_kph+VVMC_RFWhlSpeedRollAve_kph)/TWO_FLOAT}
    (junction 41) -> (junction 52) [order 2]
    (junction 69) -> (junction 47) : {VVMC_FrontRearSlipRatioCtrl_flg = FALSE}
    (junction 52) -> (junction 42) [order 1] : [VINP_LFRawWhlSpeedV_flg == TRUE]
    (junction 52) -> (junction 46) [order 2] : {VVMC_FrontAxleWhlSpeedAve_kph = VVMC_LFWhlSpeedRollAve_kph}
    (junction 42) -> (junction 49) : {VVMC_FrontAxleWhlSpeedAve_kph = VVMC_RFWhlSpeedRollAve_kph}
    (junction 46) -> (junction 54)
    (junction 49) -> (junction 46)
    (junction 54) -> (junction 92)
    (junction 92) -> (junction 85) [order 1] : [VINP_LRRawWhlSpeedV_flg == TRUE ||...
        |  VINP_RRRawWhlSpeedV_flg == TRUE]
    (junction 85) -> (junction 77) [order 1] : [VINP_LRRawWhlSpeedV_flg == TRUE &&...
        |  VINP_RRRawWhlSpeedV_flg == TRUE]
    (junction 92) -> (junction 80) [order 2] : {VVMC_RearAxleWhlSpeedAve_kph =...
        | (VVMC_LRWhlSpeedRollAve_kph+VVMC_RRWhlSpeedRollAve_kph)/TWO_FLOAT}
    (junction 85) -> (junction 89) [order 2]
    (junction 77) -> (junction 79) : {VVMC_FrontRearSlipRatioCtrl_flg = FALSE}
    (junction 89) -> (junction 84) [order 1] : [VINP_LRRawWhlSpeedV_flg == TRUE]
    (junction 89) -> (junction 82) [order 2] : {VVMC_RearAxleWhlSpeedAve_kph = VVMC_LRWhlSpeedRollAve_kph}
    (junction 84) -> (junction 78) : {VVMC_RearAxleWhlSpeedAve_kph = VVMC_RRWhlSpeedRollAve_kph}
    (junction 82) -> (junction 80)
    (junction 78) -> (junction 82)
    (junction 80) -> (junction 96)
    (junction 96) -> (junction 98) [order 1] : [abs(VVMC_RearAxleWhlSpeedAve_kph - VVMC_FrontAxleWhlSpeedAve_kph) >= KVMC_FrontRearSlipRatioTHR_kph]
    (junction 96) -> (junction 103) [order 2] : {VVMC_FrontRearSlipRatioCtrl_flg = FALSE}
    (junction 98) -> (junction 100) : {VVMC_FrontRearSlipRatioCtrl_flg = TRUE}
  data: VVMC_LFWhlSpeedRollAve_kph input single; VVMC_RFWhlSpeedRollAve_kph input single; VVMC_LRWhlSpeedRollAve_kph input single; VVMC_RRWhlSpeedRollAve_kph input single; VINP_LFRawWhlSpeedV_flg input boolean; VINP_RFRawWhlSpeedV_flg input boolean; VINP_LRRawWhlSpeedV_flg input boolean; VINP_RRRawWhlSpeedV_flg input boolean; KVMC_FrontRearSlipRatioTHR_kph input single; TRUE input boolean; VVMC_FrontRearSlipRatioCtrl_flg output boolean; FALSE input boolean; TWO_FLOAT input single; VVMC_FrontAxleWhlSpeedAve_kph local single; ZERO_FLOAT input single; VVMC_RearAxleWhlSpeedAve_kph local single

== stateflow chart vmc/VMC/VMC/IMU/IMU sensing result /RollingAverage ==
  state RollingAverage
    (default) -> (junction 2) : {VVMC_RollAveCount_enum = ONE_INT}
    RollingAverage -> (junction 2)
    (junction 2) -> (junction 3) : {VVMC_RollAve_raw32 = ZERO_FLOAT}
    (junction 3) -> (junction 100) [order 1] : [VVMC_RollAveCount_enum < KVMC_RollAveLevel_enum]
    (junction 3) -> (junction 37) [order 2]
    (junction 100) -> (junction 5) : {% Memory
        |  VVMC_Memory_raw32[VVMC_RollAveCount_enum] = VINP_INPData_raw32;
        |
        |  % Memory Shift Counter
        |  VVMC_ShiftCount_enum = ONE_INT}
    (junction 5) -> (junction 7) [order 2]
    (junction 5) -> (junction 6) [order 1] : [VVMC_ShiftCount_enum <= VVMC_RollAveCount_enum]
    (junction 7) -> (junction 8) : {% Rolling Average
        |  VVMC_RollAve_raw32 = VVMC_RollAve_raw32 / VVMC_RollAveCount_enum;
        |
        |  % Rolling Average Counter
        |  VVMC_RollAveCount_enum++}
    (junction 35) -> (junction 5) : {VVMC_ShiftCount_enum++}
    (junction 6) -> (junction 36) : {% Rolling Average Sum
        |  VVMC_RollAve_raw32 = VVMC_RollAve_raw32 + VVMC_Memory_raw32[VVMC_ShiftCount_enum];
        |  }
    (junction 36) -> (junction 35)
    (junction 37) -> (junction 76) [order 1] : [VVMC_RollAveCount_enum == KVMC_RollAveLevel_enum]
    (junction 76) -> (junction 47)
    (junction 37) -> (junction 60) [order 2]
    (junction 78) -> (junction 76)
    (junction 47) -> (junction 30) : {% Memory
        |  VVMC_Memory_raw32[VVMC_RollAveCount_enum] = VINP_INPData_raw32;
        |
        |  % Memory Shift Counter
        |  VVMC_ShiftCount_enum = ONE_INT;
        | }
    (junction 60) -> (junction 62) [order 1] : [VVMC_RollAveCount_enum > KVMC_RollAveLevel_enum]
    (junction 60) -> (junction 39) [order 2]
    (junction 62) -> (junction 66) : {VVMC_MemoryShiftCount_enum = ONE_INT}
    (junction 30) -> (junction 48) [order 2]
    (junction 30) -> (junction 22) [order 1] : [VVMC_ShiftCount_enum <= VVMC_RollAveCount_enum]
    (junction 48) -> (junction 45) : {% Rolling Average
        |  VVMC_RollAve_raw32 = VVMC_RollAve_raw32 / VVMC_RollAveCount_enum;
        |
        |  % Memory Shift Counter
        |  VVMC_ShiftCount_enum = ONE_INT}
    (junction 14) -> (junction 30) : {VVMC_ShiftCount_enum++}
    (junction 22) -> (junction 25) : {% Rolling Average Sum
        |  VVMC_RollAve_raw32 = VVMC_RollAve_raw32 + VVMC_Memory_raw32[VVMC_ShiftCount_enum]}
    (junction 66) -> (junction 82) [order 2]
    (junction 66) -> (junction 69) [order 1] : [VVMC_MemoryShiftCount_enum < VVMC_RollAveCount_enum]
    (junction 82) -> (junction 80) : {VVMC_RollAveCount_enum = KVMC_RollAveLevel_enum}
    (junction 73) -> (junction 66) : {VVMC_MemoryShiftCount_enum++}
    (junction 69) -> (junction 71) : {VVMC_Memory_raw32[VVMC_MemoryShiftCount_enum] =...
        |  VVMC_Memory_raw32[VVMC_RollAveCount_enum - KVMC_RollAveLevel_enum + VVMC_MemoryShiftCount_enum]}
    (junction 25) -> (junction 14)
    (junction 71) -> (junction 73)
    (junction 80) -> (junction 78)
    (junction 45) -> (junction 39) [order 2]
    (junction 45) -> (junction 15) [order 1] : [VVMC_ShiftCount_enum < VVMC_RollAveCount_enum]
    (junction 41) -> (junction 45) : { VVMC_ShiftCount_enum++}
    (junction 15) -> (junction 38) : {% Gy Memory Shift
        |  VVMC_Memory_raw32[VVMC_ShiftCount_enum] = VVMC_Memory_raw32[VVMC_ShiftCount_enum + ONE_INT]}
    (junction 38) -> (junction 41)
  data: KVMC_RollAveLevel_enum input uint8; VVMC_ShiftCount_enum local uint8; VVMC_RollAveCount_enum local uint8; VVMC_Memory_raw32 local single size=256; ZERO_FLOAT input single; ONE_INT input uint8; VVMC_RollAve_raw32 output single; VINP_INPData_raw32 input single; VVMC_MemoryShiftCount_enum local uint8

== stateflow chart vmc/VMC/VMC/SafetyControl/SafetyControlJudgement/RearWheelSlipRatio/FrontRearSlipRatioJudgement ==
  state RearWheelSlipRatioJudgement
    (default) -> (junction 14) : {VVMC_RearWhlSlipRatioCtrl_flg = FALSE}
    RearWheelSlipRatioJudgement -> (junction 14)
    (junction 14) -> (junction 85) [order 1] : [VINP_LRRawWhlSpeedV_flg == TRUE ||...
        |  VINP_RRRawWhlSpeedV_flg == TRUE]
    (junction 14) -> (junction 96) [order 2]
    (junction 85) -> (junction 105) : {VVMC_RearWhlSlipRatioCtrl_flg = FALSE}
    (junction 96) -> (junction 98) [order 1] : [abs(VVMC_LRWhlSpeedRollAve_kph - VVMC_RRWhlSpeedRollAve_kph) >= KVMC_RearWhlSlipRatioTHR_kph]
    (junction 96) -> (junction 103) [order 2] : {VVMC_RearWhlSlipRatioCtrl_flg = FALSE}
    (junction 98) -> (junction 100) : {VVMC_RearWhlSlipRatioCtrl_flg = TRUE}
  data: VVMC_LRWhlSpeedRollAve_kph input single; VVMC_RRWhlSpeedRollAve_kph input single; VINP_LRRawWhlSpeedV_flg input boolean; VINP_RRRawWhlSpeedV_flg input boolean; KVMC_RearWhlSlipRatioTHR_kph input single; TRUE input boolean; VVMC_RearWhlSlipRatioCtrl_flg output boolean; FALSE input boolean

== stateflow chart vmc/VMC/VMC/SafetyControl/SafetyControlJudgement/SingleWheelSlipRatio/SingleWheelSlipRatioJudgement ==
  state SingleWheelSlipRatioJudgement
    (default) -> (junction 14) : {VVMC_SingleWhlSlipRatioCtrl_flg = FALSE}
    SingleWheelSlipRatioJudgement -> (junction 14)
    (junction 14) -> (junction 105) [order 1] : [VINP_LFRawWhlSpeedV_flg == FALSE]
    (junction 105) -> (junction 117) [order 1] : [abs(VINP_VehSpeed_kph - VVMC_LFWhlSpeedRollAve_kph) >= KVMC_SingleWhlSlipRatioTHR_kph]
    (junction 14) -> (junction 121) [order 2]
    (junction 105) -> (junction 119) [order 2]
    (junction 117) -> (junction 107) : {VVMC_SingleWhlSlipRatioCtrl_flg = TRUE}
    (junction 119) -> (junction 121)
    (junction 121) -> (junction 134)
    (junction 134) -> (junction 130) [order 1] : [VINP_RFRawWhlSpeedV_flg == FALSE]
    (junction 130) -> (junction 125) [order 1] : [abs(VINP_VehSpeed_kph - VVMC_RFWhlSpeedRollAve_kph) >= KVMC_SingleWhlSlipRatioTHR_kph]
    (junction 134) -> (junction 127) [order 2]
    (junction 130) -> (junction 132) [order 2]
    (junction 125) -> (junction 131) : {VVMC_SingleWhlSlipRatioCtrl_flg = TRUE}
    (junction 132) -> (junction 127)
    (junction 127) -> (junction 143)
    (junction 143) -> (junction 149) [order 1] : [VINP_LRRawWhlSpeedV_flg == FALSE]
    (junction 149) -> (junction 144) [order 1] : [abs(VINP_VehSpeed_kph - VVMC_LRWhlSpeedRollAve_kph) >= KVMC_SingleWhlSlipRatioTHR_kph]
    (junction 143) -> (junction 137) [order 2]
    (junction 149) -> (junction 146) [order 2]
    (junction 144) -> (junction 148) : {VVMC_SingleWhlSlipRatioCtrl_flg = TRUE}
    (junction 146) -> (junction 137)
    (junction 137) -> (junction 154)
    (junction 154) -> (junction 153) [order 1] : [VINP_RRRawWhlSpeedV_flg == FALSE]
    (junction 153) -> (junction 150) [order 1] : [abs(VINP_VehSpeed_kph - VVMC_RRWhlSpeedRollAve_kph) >= KVMC_SingleWhlSlipRatioTHR_kph]
    (junction 154) -> (junction 169) [order 2]
    (junction 153) -> (junction 152) [order 2]
    (junction 150) -> (junction 155) : {VVMC_SingleWhlSlipRatioCtrl_flg = TRUE}
    (junction 152) -> (junction 169)
    (junction 169) -> (junction 157)
    (junction 157) -> (junction 163) [order 1] : [(VINP_LFRawWhlSpeedV_flg == TRUE &&...
        |   VINP_RFRawWhlSpeedV_flg == TRUE) ||...
        |  (VINP_LRRawWhlSpeedV_flg == TRUE &&...
        |   VINP_RRRawWhlSpeedV_flg == TRUE)]
    (junction 157) -> (junction 167) [order 2] : {VVMC_SingleWhlSlipRatioCtrl_flg = FALSE}
    (junction 163) -> (junction 165) : {VVMC_SingleWhlSlipRatioCtrl_flg = TRUE}
  data: VINP_VehSpeed_kph input single; VVMC_LFWhlSpeedRollAve_kph input single; VVMC_RFWhlSpeedRollAve_kph input single; VVMC_LRWhlSpeedRollAve_kph input single; VVMC_RRWhlSpeedRollAve_kph input single; VINP_LFRawWhlSpeedV_flg input boolean; VINP_RFRawWhlSpeedV_flg input boolean; VINP_LRRawWhlSpeedV_flg input boolean; VINP_RRRawWhlSpeedV_flg input boolean; KVMC_SingleWhlSlipRatioTHR_kph input single; TRUE input boolean; VVMC_SingleWhlSlipRatioCtrl_flg output boolean; FALSE input boolean

== stateflow chart vmc/VMC/VMC/SpeedArbitration/Response Gain/Response Gain ==
  state ResponseGain
    (default) -> (junction 81) : {VVMC_JerkPCT_pct = ZERO_FLOAT;
        |  VVMC_LimitPCT_pct = ZERO_FLOAT}
    ResponseGain -> (junction 81)
    (junction 81) -> (junction 73) [order 1] : [VVMC_FeatArbitrSta_enum == ENUM_FEATARBITRSTA_DISC ||...
        |  VVMC_FeatArbitrSta_enum == ENUM_FEATARBITRSTA_CC ||...
        |  VVMC_FeatArbitrSta_enum == ENUM_FEATARBITRSTA_MSA ||...
        |  VVMC_FeatArbitrSta_enum == ENUM_FEATARBITRSTA_ACCDISC]
    (junction 73) -> (junction 75) [order 1] : [VDSC_DISCTurn_flg == ENUM_DISCTURN_ACTIVE ||...
        | (VVMC_FeatArbitrSta_enum == ENUM_FEATARBITRSTA_MSA &&...
        |  KVMC_MSAResponseAGSV_flg == TRUE)]
    (junction 81) -> (junction 92) [order 2] : {VVMC_JerkPCT_pct = ZERO_FLOAT;
        |  VVMC_LimitPCT_pct = ZERO_FLOAT}
    (junction 73) -> (junction 77) [order 2] : {VVMC_JerkPCT_pct = VVMC_SoftJerkPCT_pct;
        |  VVMC_LimitPCT_pct = VVMC_SoftLimitPCT_pct}
    (junction 75) -> (junction 78) : {VVMC_JerkPCT_pct = VVMC_AggressJerkPCT_pct;
        |  VVMC_LimitPCT_pct = VVMC_AggressLimitPCT_pct}
  data: VDSC_DISCTurn_flg input uint8; VVMC_FeatArbitrSta_enum input uint8; VVMC_JerkPCT_pct output single; VVMC_LimitPCT_pct output single; VVMC_SoftJerkPCT_pct input single; VVMC_AggressJerkPCT_pct input single; VVMC_SoftLimitPCT_pct input single; VVMC_AggressLimitPCT_pct input single; ENUM_FEATARBITRSTA_DISC input uint8; ENUM_FEATARBITRSTA_CC input; ZERO_FLOAT input single; ENUM_DISCTURN_ACTIVE input uint8; ENUM_FEATARBITRSTA_ACCDISC input uint8; ENUM_FEATARBITRSTA_MSA input; TRUE input; KVMC_MSAResponseAGSV_flg input; ENUM_FEATARBITRSTA_ACC parameter

== stateflow chart vmc/VMC/VMC/SpeedArbitration/Feature Status Confirm/Feature Status Confirm ==
  state FeatStaConfrim
    (default) -> (junction 197) : {VVMC_FeatStaConfirm_enum = ENUM_FEATSTACFM_INACTIVE}
    FeatStaConfrim -> (junction 197)
    (junction 197) -> (junction 203) [order 1] : [VVMC_VMCAEBCtrlAvail_flg == ENUM_VMCAEBCTRLAVAIL_AVAILABLE &&...
        | (VINP_ADASAEBSta_enum == ENUM_ADASAEBSTA_ACTIVE ||...
        |  VINP_ADASAEBReq_enum ~= ENUM_ADASAEBREQ_NOREQUEST)]
    (junction 197) -> (junction 200) [order 2]
    (junction 203) -> (junction 202) : {VVMC_FeatStaConfirm_enum = ENUM_FEATSTACFM_AEB}
    (junction 200) -> (junction 208) [order 1] : [VVMC_VMCACCCtrlAvail_flg == ENUM_VMCACCCTRLAVAIL_AVAILABLE &&...
        | (VDSC_DISCSta_enum == ENUM_DISCSTA_ACTIVE || VDSC_PreACC_flg)]
    (junction 208) -> (junction 210) [order 1] : [VINP_ADASACCSta_enum == ENUM_ADASACCSTA_ACTIVE ||...
        |  VINP_ADASACCSta_enum == ENUM_ADASACCSTA_SHUTOFF ||...
        |  VINP_ADASACCSta_enum == ENUM_ADASACCSTA_OVERRIDE]
    (junction 200) -> (junction 232) [order 2]
    (junction 208) -> (junction 214) [order 2]
    (junction 210) -> (junction 212) : {VVMC_FeatStaConfirm_enum = ENUM_FEATSTACFM_ACCDISC}
    (junction 214) -> (junction 216) [order 1] : [(VVMC_CCCtrlSta_enum == ENUM_CCCRLSTA_ACTIVE ||...
        |   VVMC_CCCtrlSta_enum == ENUM_CCCRLSTA_OVERRIDE) &&...
        |  VVMC_VMCCCCtrlAvail_flg == ENUM_VMCCCCTRLAVAIL_AVAILABLE]
    (junction 214) -> (junction 222) [order 2]
    (junction 216) -> (junction 218) : {VVMC_FeatStaConfirm_enum = ENUM_FEATSTACFM_CCDISC}
    (junction 222) -> (junction 224) [order 1] : [(VVMC_MSACtrlSta_enum == ENUM_MSACRLSTA_ACTIVE ||...
        |   VVMC_MSACtrlSta_enum == ENUM_MSACRLSTA_OVERRIDE) &&...
        |  VVMC_VMCMSACtrlAvail_flg == ENUM_VMCMSACTRLAVAIL_AVAILABLE]
    (junction 222) -> (junction 229) [order 2] : {VVMC_FeatStaConfirm_enum = ENUM_FEATSTACFM_DISC}
    (junction 224) -> (junction 221) : {VVMC_FeatStaConfirm_enum = ENUM_FEATSTACFM_DISCMSA}
    (junction 232) -> (junction 234) [order 1] : [VVMC_VMCACCCtrlAvail_flg == ENUM_VMCACCCTRLAVAIL_AVAILABLE &&...
        | (VINP_ADASACCSta_enum == ENUM_ADASACCSTA_ACTIVE ||...
        |  VINP_ADASACCSta_enum == ENUM_ADASACCSTA_OVERRIDE ||...
        |  VINP_ADASACCSta_enum == ENUM_ADASACCSTA_SHUTOFF)]
    (junction 232) -> (junction 238) [order 2]
    (junction 234) -> (junction 236) : {VVMC_FeatStaConfirm_enum = ENUM_FEATSTACFM_ACC}
    (junction 238) -> (junction 240) [order 1] : [(VVMC_CCCtrlSta_enum == ENUM_CCCRLSTA_ACTIVE ||...
        |   VVMC_CCCtrlSta_enum == ENUM_CCCRLSTA_OVERRIDE) &&...
        |  VVMC_VMCCCCtrlAvail_flg == ENUM_VMCCCCTRLAVAIL_AVAILABLE]
    (junction 238) -> (junction 250) [order 2]
    (junction 240) -> (junction 244) : {VVMC_FeatStaConfirm_enum = ENUM_FEATSTACFM_CC}
    (junction 250) -> (junction 249) [order 1] : [(VVMC_MSACtrlSta_enum == ENUM_MSACRLSTA_ACTIVE ||...
        |   VVMC_MSACtrlSta_enum == ENUM_MSACRLSTA_OVERRIDE) &&...
        |  VVMC_VMCMSACtrlAvail_flg == ENUM_VMCMSACTRLAVAIL_AVAILABLE]
    (junction 250) -> (junction 252) [order 2] : {VVMC_FeatStaConfirm_enum = ENUM_FEATSTACFM_INACTIVE}
    (junction 249) -> (junction 248) : {VVMC_FeatStaConfirm_enum = ENUM_FEATSTACFM_MSA}
  data: VVMC_VMCCCCtrlAvail_flg input boolean; ENUM_VMCCCCTRLAVAIL_AVAILABLE input uint8; VVMC_VMCMSACtrlAvail_flg input boolean; ENUM_VMCMSACTRLAVAIL_AVAILABLE input uint8; VVMC_VMCAEBCtrlAvail_flg input boolean; ENUM_VMCAEBCTRLAVAIL_AVAILABLE input uint8; VVMC_VMCACCCtrlAvail_flg input boolean; ENUM_VMCACCCTRLAVAIL_AVAILABLE input uint8; VINP_ADASAEBSta_enum input uint8; VDSC_DISCSta_enum input uint8; VINP_ADASACCSta_enum input uint8; VVMC_CCCtrlSta_enum input uint8; VVMC_FeatStaConfirm_enum output uint8; VVMC_MSACtrlSta_enum input uint8; ENUM_FEATSTACFM_INACTIVE input uint8; ENUM_FEATSTACFM_AEB input uint8; ENUM_FEATSTACFM_ACC input uint8; ENUM_FEATSTACFM_CC input uint8; ENUM_FEATSTACFM_DISC input uint8; ENUM_FEATSTACFM_MSA input uint8; ENUM_FEATSTACFM_ACCDISC input uint8; ENUM_FEATSTACFM_CCDISC input uint8; ENUM_FEATSTACFM_DISCMSA input uint8; ENUM_ADASAEBSTA_ACTIVE input uint8; ENUM_ADASACCSTA_ACTIVE input uint8; ENUM_ADASACCSTA_SHUTOFF input uint8; ENUM_CCCRLSTA_ACTIVE input uint8; ENUM_MSACRLSTA_ACTIVE input uint8; ENUM_DISCSTA_ACTIVE input uint8; ENUM_ADASACCSTA_OVERRIDE input uint8; VINP_ADASAEBReq_enum input uint8; ENUM_ADASAEBREQ_NOREQUEST input uint8; ENUM_CCCRLSTA_OVERRIDE input; ENUM_MSACRLSTA_OVERRIDE input; VDSC_PreACC_flg input
